simulink model "ex8"  (Simulink 8.1)
settings: Solver=ode45  StartTime=0.0  StopTime=10.0  RelTol=1e-3
values from neighbouring files (symbols this model uses):
  Gam = [T^2/2; T]    [ex8_init.m]
  H = [1 0]    [ex8_init.m]    (also in ss512_init.m = [1 0 0 0])
  K = acker(Phi, Gam, p)    [ex8_init.m]    (also in myacker.m = en*(W\alpha); ss1_init.m = myacker(Phi, Gamma, z))
  Lp = acker(Phi', H', p)'    [ex8_init.m]    (also in ss512_init.m = acker(Phi', H', z3)')
  Phi = [1 T; 0 1]    [ex8_init.m]
  T = 0.1    [ex8_init.m]    (also in ss1_init.m; ss512_init.m = 0.4; ss51_init.m = 0.4)
  x1 = [1; 0]    [ex8_init.m]    (also in ss1_init.m = [1; 1]; ss512_init.m = [1; 0; 0; 0]; ss51_init.m = [1; 0; 0; 0])
settings Model: Creator=jmahler  LastModifiedBy=jmahler
settings DataIOCC: SignalLoggingSaveFormat=Dataset
settings OptimizationCC: ExpressionDepthLimit=128
settings DebuggingCC: FcnCallInpInsideContextMsg=EnableAllAsError
settings GRTTargetCC: CombineOutputUpdateFcns=on  GRTInterface=off

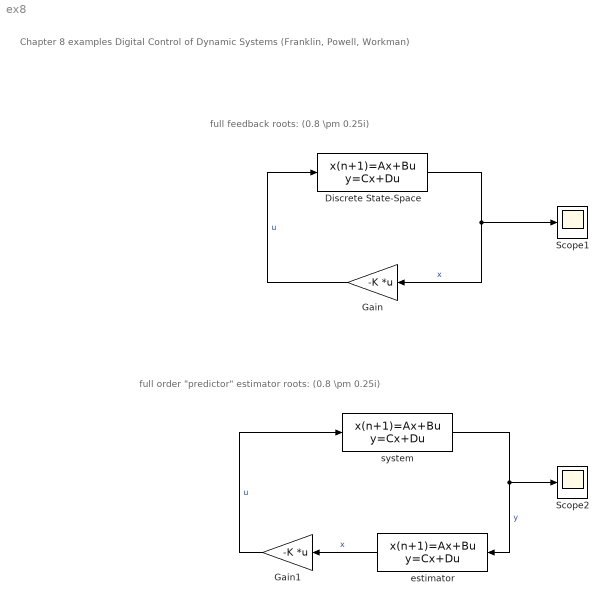
== system ex8 ==
  note: Chapter 8 examples
      | Digital Control of Dynamic Systems (Franklin, Powell, Workman)
  note: full feedback
      | roots: (0.8 \pm 0.25i)
  note: full order "predictor" estimator
      | roots: (0.8 \pm 0.25i)
  Discrete State-Space : DiscreteStateSpace  A=Phi  B=Gam  C=eye(2)  D=[0; 0]  X0=x1  SampleTime=T
  Gain : Gain  Gain=-K  Multiplication=Matrix(K*u)  SampleTime=T
  Gain1 : Gain  Gain=-K  Multiplication=Matrix(K*u)  SampleTime=T
  Scope1 : Scope
  Scope2 : Scope
  estimator : DiscreteStateSpace  A=(Phi - Gam*K - Lp*H)  B=Lp  C=eye(2)  D=[0; 0]  X0=x1  SampleTime=T
  system : DiscreteStateSpace  A=Phi  B=Gam  C=H  D=[0]  X0=x1  SampleTime=T
  wires:
  Discrete State-Space/1 -> Scope1/1, Gain/1  "x"
  Gain/1 -> Discrete State-Space/1  "u"
  system/1 -> Scope2/1, estimator/1  "y"
  Gain1/1 -> system/1  "u"
  estimator/1 -> Gain1/1  "x"
